simulink model "AME556_Project_Task4_v2"  (R2024b)
settings: Solver=VariableStepAuto  StartTime=0.0  StopTime=5  FixedStep=0.0005  RelTol=1e-3  AbsTol=1e-3
InitFcn:
  | global params;
  | 
  | % Mass and geometry
  | params.m = 0.25;
  | params.l = 0.22;
  | params.mb = 8;
  | params.a = 0.25;
  | params.b = 0.15;
  | params.g = [0; 9.81; 0];
  | 
  | % Moment of inerita
  | Il_zz = params.m * params.l^2 / 12;
  | Ib_xx = params.mb * params.a^2 / 12;
  | Ib_yy = params.mb * params.b^2 / 12;
  | Ib_zz = params.mb * (params.a^2 + params.b^2) / 12;
  | params.Ib = diag([Ib_xx Ib_yy Ib_zz]);
  | 
  | % Spatial contact force parameters
  | Kp_g = 1e5;
  | Kd_g = 1e3;
  | 
  | % Ground contact positions
  | params.P1 = [0.0197; 0.0022; 0];
  | params.P2 = [0.1838; 0.0041; 0];
  | 
  | % State variables
  | q0 = [0.1; 0.45; 0; -pi/3; pi/2; -pi/6; pi/2]; % Initial states (before landing)
  | params.p_d = [0; 0.5; 0]; % Desired positions (after standing): [x_d; y_d; z_d];
  | params.theta_d = 0; % Desired angle
values from neighbouring files (symbols this model uses):
  dt = 0.04    [AME556_Project_Task4_Setup.m]
  l = 2    [AME556_Project_Task4_Setup.m]
  N = 10    [AME556_Project_Task4_Setup.m]
undefined symbols (not defined in the file or in its folder): P1_world0, P2_world0, X, Y, Z
libraries: sm_lib x37, nesl_utility x23
(part 2 of 2)

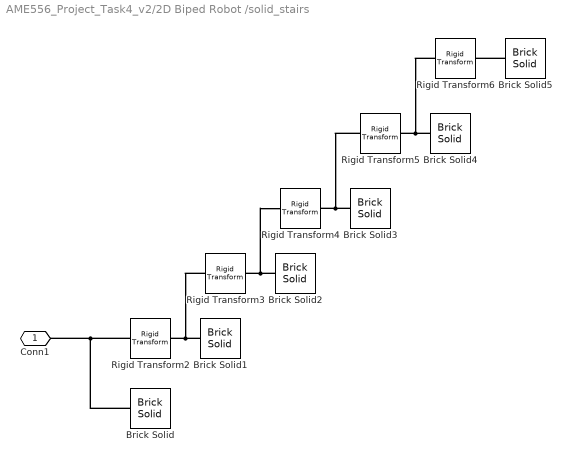
== system AME556_Project_Task4_v2/2D Biped Robot /solid_stairs ==
  Brick Solid : sm_lib/Body Elements/Brick Solid  BrickDimensions=[x_grid(end) y_grid(end) 0.1 ]  BrickDimensionsUnits=m  ExportEntireGeometry=off  InertiaType=CalculateFromGeometry  BasedOnType=Density  Density=1000  DensityUnits=kg/m^3  Mass=1  MassUnits=kg  CenterOfMass=[0 0 0]  CenterOfMassUnits=m  MomentsOfInertia=[1 1 1]  MomentsOfInertiaUnits=kg*m^2  ProductsOfInertia=[0 0 0]  ProductsOfInertiaUnits=kg*m^2  GraphicType=FromGeometry  MarkerShape=Sphere  MarkerSize=10  GraphicVisPropType=SimpleVisualProperties  GraphicDiffuseColor=stairsColor  GraphicOpacity=1  GraphicSpecularColor=[0.5 0.5 0.5 1.0]  GraphicAmbientColor=[0.15 0.15 0.15 1.0]  GraphicEmissiveColor=[0.0 0.0 0.0 1.0]  GraphicShininess=75  DoExposeReferenceFrame=on  SerializedFrames=<Frames><Frame><Id>Frame1</Id><Value><Name>F1</Name><Origin><Source>GeometricFeature</Source><FeatureName>-x -y +z point</FeatureName></Origin><PrimaryAxis><DefinedDirection>+Z</DefinedDirection><Source>ReferenceFrame</Source><SourceDirection>+Z</SourceDirection><FeatureName></FeatureName></PrimaryAxis><SecondaryAxis><DefinedDirection>+X</DefinedDirection><Source>ReferenceFrame</Source><SourceDirection>+X</SourceDirection><FeatureName></FeatureName></SecondaryAxis></Value></Frame></Frames>
  Brick Solid1 : sm_lib/Body Elements/Brick Solid  BrickDimensions=[x_grid(end) 0.8+l 0.1 ]  BrickDimensionsUnits=m  ExportEntireGeometry=off  InertiaType=CalculateFromGeometry  BasedOnType=Density  Density=1000  DensityUnits=kg/m^3  Mass=1  MassUnits=kg  CenterOfMass=[0 0 0]  CenterOfMassUnits=m  MomentsOfInertia=[1 1 1]  MomentsOfInertiaUnits=kg*m^2  ProductsOfInertia=[0 0 0]  ProductsOfInertiaUnits=kg*m^2  GraphicType=FromGeometry  MarkerShape=Sphere  MarkerSize=10  GraphicVisPropType=SimpleVisualProperties  GraphicDiffuseColor=stairsColor  GraphicOpacity=1  GraphicSpecularColor=[0.5 0.5 0.5 1.0]  GraphicAmbientColor=[0.15 0.15 0.15 1.0]  GraphicEmissiveColor=[0.0 0.0 0.0 1.0]  GraphicShininess=75  DoExposeReferenceFrame=on  SerializedFrames=<Frames><Frame><Id>Frame1</Id><Value><Name>F1</Name><Origin><Source>GeometricFeature</Source><FeatureName>-x -y -z point</FeatureName></Origin><PrimaryAxis><DefinedDirection>+Z</DefinedDirection><Source>ReferenceFrame</Source><SourceDirection>+Z</SourceDirection><FeatureName></FeatureName></PrimaryAxis><SecondaryAxis><DefinedDirection>+X</DefinedDirection><Source>ReferenceFrame</Source><SourceDirection>+X</SourceDirection><FeatureName></FeatureName></SecondaryAxis></Value></Frame></Frames>
  Brick Solid2 : sm_lib/Body Elements/Brick Solid  BrickDimensions=[x_grid(end) 0.6+l 0.1 ]  BrickDimensionsUnits=m  ExportEntireGeometry=off  InertiaType=CalculateFromGeometry  BasedOnType=Density  Density=1000  DensityUnits=kg/m^3  Mass=1  MassUnits=kg  CenterOfMass=[0 0 0]  CenterOfMassUnits=m  MomentsOfInertia=[1 1 1]  MomentsOfInertiaUnits=kg*m^2  ProductsOfInertia=[0 0 0]  ProductsOfInertiaUnits=kg*m^2  GraphicType=FromGeometry  MarkerShape=Sphere  MarkerSize=10  GraphicVisPropType=SimpleVisualProperties  GraphicDiffuseColor=stairsColor  GraphicOpacity=1  GraphicSpecularColor=[0.5 0.5 0.5 1.0]  GraphicAmbientColor=[0.15 0.15 0.15 1.0]  GraphicEmissiveColor=[0.0 0.0 0.0 1.0]  GraphicShininess=75  DoExposeReferenceFrame=on  SerializedFrames=<Frames><Frame><Id>Frame1</Id><Value><Name>F1</Name><Origin><Source>GeometricFeature</Source><FeatureName>-x -y -z point</FeatureName></Origin><PrimaryAxis><DefinedDirection>+Z</DefinedDirection><Source>ReferenceFrame</Source><SourceDirection>+Z</SourceDirection><FeatureName></FeatureName></PrimaryAxis><SecondaryAxis><DefinedDirection>+X</DefinedDirection><Source>ReferenceFrame</Source><SourceDirection>+X</SourceDirection><FeatureName></FeatureName></SecondaryAxis></Value></Frame></Frames>
  Brick Solid3 : sm_lib/Body Elements/Brick Solid  BrickDimensions=[x_grid(end) 0.4+l 0.1 ]  BrickDimensionsUnits=m  ExportEntireGeometry=off  InertiaType=CalculateFromGeometry  BasedOnType=Density  Density=1000  DensityUnits=kg/m^3  Mass=1  MassUnits=kg  CenterOfMass=[0 0 0]  CenterOfMassUnits=m  MomentsOfInertia=[1 1 1]  MomentsOfInertiaUnits=kg*m^2  ProductsOfInertia=[0 0 0]  ProductsOfInertiaUnits=kg*m^2  GraphicType=FromGeometry  MarkerShape=Sphere  MarkerSize=10  GraphicVisPropType=SimpleVisualProperties  GraphicDiffuseColor=stairsColor  GraphicOpacity=1  GraphicSpecularColor=[0.5 0.5 0.5 1.0]  GraphicAmbientColor=[0.15 0.15 0.15 1.0]  GraphicEmissiveColor=[0.0 0.0 0.0 1.0]  GraphicShininess=75  DoExposeReferenceFrame=on  SerializedFrames=<Frames><Frame><Id>Frame1</Id><Value><Name>F1</Name><Origin><Source>GeometricFeature</Source><FeatureName>-x -y -z point</FeatureName></Origin><PrimaryAxis><DefinedDirection>+Z</DefinedDirection><Source>ReferenceFrame</Source><SourceDirection>+Z</SourceDirection><FeatureName></FeatureName></PrimaryAxis><SecondaryAxis><DefinedDirection>+X</DefinedDirection><Source>ReferenceFrame</Source><SourceDirection>+X</SourceDirection><FeatureName></FeatureName></SecondaryAxis></Value></Frame></Frames>
  Brick Solid4 : sm_lib/Body Elements/Brick Solid  BrickDimensions=[x_grid(end) 0.2+l 0.1 ]  BrickDimensionsUnits=m  ExportEntireGeometry=off  InertiaType=CalculateFromGeometry  BasedOnType=Density  Density=1000  DensityUnits=kg/m^3  Mass=1  MassUnits=kg  CenterOfMass=[0 0 0]  CenterOfMassUnits=m  MomentsOfInertia=[1 1 1]  MomentsOfInertiaUnits=kg*m^2  ProductsOfInertia=[0 0 0]  ProductsOfInertiaUnits=kg*m^2  GraphicType=FromGeometry  MarkerShape=Sphere  MarkerSize=10  GraphicVisPropType=SimpleVisualProperties  GraphicDiffuseColor=stairsColor  GraphicOpacity=1  GraphicSpecularColor=[0.5 0.5 0.5 1.0]  GraphicAmbientColor=[0.15 0.15 0.15 1.0]  GraphicEmissiveColor=[0.0 0.0 0.0 1.0]  GraphicShininess=75  DoExposeReferenceFrame=on  SerializedFrames=<Frames><Frame><Id>Frame1</Id><Value><Name>F1</Name><Origin><Source>GeometricFeature</Source><FeatureName>-x -y -z point</FeatureName></Origin><PrimaryAxis><DefinedDirection>+Z</DefinedDirection><Source>ReferenceFrame</Source><SourceDirection>+Z</SourceDirection><FeatureName></FeatureName></PrimaryAxis><SecondaryAxis><DefinedDirection>+X</DefinedDirection><Source>ReferenceFrame</Source><SourceDirection>+X</SourceDirection><FeatureName></FeatureName></SecondaryAxis></Value></Frame></Frames>
  Brick Solid5 : sm_lib/Body Elements/Brick Solid  BrickDimensions=[x_grid(end) l 0.1 ]  BrickDimensionsUnits=m  ExportEntireGeometry=off  InertiaType=CalculateFromGeometry  BasedOnType=Density  Density=1000  DensityUnits=kg/m^3  Mass=1  MassUnits=kg  CenterOfMass=[0 0 0]  CenterOfMassUnits=m  MomentsOfInertia=[1 1 1]  MomentsOfInertiaUnits=kg*m^2  ProductsOfInertia=[0 0 0]  ProductsOfInertiaUnits=kg*m^2  GraphicType=FromGeometry  MarkerShape=Sphere  MarkerSize=10  GraphicVisPropType=SimpleVisualProperties  GraphicDiffuseColor=stairsColor  GraphicOpacity=1  GraphicSpecularColor=[0.5 0.5 0.5 1.0]  GraphicAmbientColor=[0.15 0.15 0.15 1.0]  GraphicEmissiveColor=[0.0 0.0 0.0 1.0]  GraphicShininess=75  DoExposeReferenceFrame=on  SerializedFrames=<Frames><Frame><Id>Frame1</Id><Value><Name>F1</Name><Origin><Source>GeometricFeature</Source><FeatureName>-x -y -z point</FeatureName></Origin><PrimaryAxis><DefinedDirection>+Z</DefinedDirection><Source>ReferenceFrame</Source><SourceDirection>+Z</SourceDirection><FeatureName></FeatureName></PrimaryAxis><SecondaryAxis><DefinedDirection>+X</DefinedDirection><Source>ReferenceFrame</Source><SourceDirection>+X</SourceDirection><FeatureName></FeatureName></SecondaryAxis></Value></Frame></Frames>
  Rigid Transform2 : sm_lib/Frames and Transforms/Rigid Transform  RotationMethod=None  FollAlignAxisA=+X  BaseAlignAxisA=+Z  FollAlignAxisB=+Y  BaseAlignAxisB=+X  RotationStandardAxis=+Z  RotationAngle=0  RotationAngleUnits=deg  RotationArbitraryAxis=[0 0 1]  RotationSequenceAxes=FollowerAxes  RotationSequence=XYX  RotationSequenceAngles=[0 0 0]  RotationSequenceAnglesUnits=deg  RotationMatrix=[1 0 0;0 1 0;0 0 1]  Quaternion=[1 0 0 0]  TranslationMethod=StandardAxis  TranslationCartesianOffset=[0 0 0]  TranslationCartesianOffsetUnits=m  TranslationStandardAxis=+Y  TranslationStandardOffset=l  TranslationStandardOffsetUnits=m  TranslationROffset=0  TranslationROffsetUnits=m  TranslationThetaOffset=0  TranslationThetaOffsetUnits=deg  TranslationZOffset=0  TranslationZOffsetUnits=m
  Rigid Transform{3..6} (4 alike) : sm_lib/Frames and Transforms/Rigid Transform  RotationMethod=None  FollAlignAxisA=+X  BaseAlignAxisA=+Z  FollAlignAxisB=+Y  BaseAlignAxisB=+X  RotationStandardAxis=+Z  RotationAngle=0  RotationAngleUnits=deg  RotationArbitraryAxis=[0 0 1]  RotationSequenceAxes=FollowerAxes  RotationSequence=XYX  RotationSequenceAngles=[0 0 0]  RotationSequenceAnglesUnits=deg  RotationMatrix=[1 0 0;0 1 0;0 0 1]  Quaternion=[1 0 0 0]  TranslationMethod=Cartesian  TranslationCartesianOffset=[0 0.2 0.1]  TranslationCartesianOffsetUnits=m  TranslationStandardAxis=+Y  TranslationStandardOffset=l  TranslationStandardOffsetUnits=m  TranslationROffset=0  TranslationROffsetUnits=m  TranslationThetaOffset=0  TranslationThetaOffsetUnits=deg  TranslationZOffset=0  TranslationZOffsetUnits=m
  Conn1 : PMIOPort  Side=Left
  connections:
  Brick Solid3/LConn1 -- Rigid Transform5/LConn1 -- Rigid Transform4/RConn1
  Brick Solid2/LConn1 -- Rigid Transform4/LConn1 -- Rigid Transform3/RConn1
  Brick Solid4/LConn1 -- Rigid Transform6/LConn1 -- Rigid Transform5/RConn1
  Brick Solid/LConn1 -- Conn1/RConn1 -- Rigid Transform2/LConn1
  Brick Solid1/LConn1 -- Rigid Transform3/LConn1 -- Rigid Transform2/RConn1
  Brick Solid5/LConn1 -- Rigid Transform6/RConn1

== matlab function AME556_Project_Task4_v2/MATLAB Function ==
  data: tau_unsaturated input; tau_saturated output; saturateSwitch input
function tau_saturated = tau_saturation(tau_unsaturated, saturateSwitch)
    if saturateSwitch == 1
        tau_limits = [30, 60, 30, 60];
    
        tau_saturated = tau_unsaturated;
    
        for i = 1:length(tau_unsaturated)
            if tau_unsaturated(i) > tau_limits(i)
                tau_saturated(i) = tau_limits(i);
                warning('Tau %d (%.2f) is saturated to %d', i, tau_unsaturated(i), tau_limits(i));
            elseif tau_unsaturated(i) < -tau_limits(i)
                tau_saturated(i) = -tau_limits(i);
                warning('Tau %d (%.2f) is saturated to -%d', i, tau_unsaturated(i), tau_limits(i));
            end
        end
    else
        tau_saturated = tau_unsaturated;
    end
end

== matlab function AME556_Project_Task4_v2/Controller/Condensed MPC Controller ==
  data: p input; theta input; dp input; dtheta input; qs input; tau output; P1 input; P2 input; dP1 input; dP2 input; N input; dt input; t input
%% Function: Low Level Control

function tau = lowLevelControl(p, theta, dp, dtheta, qs, P1, P2, dP1, dP2, N, dt, t)

con = gaitSchedule(N, dt, t);
F = condensed_mpc_controller(p, theta, dp, dtheta, P1, P2, N, dt, t, con);
J = jacobianFcn(theta, qs);

tau = zeros(4, 1);
if con(1, 1) && con(2, 1)
    tau = -J' * F;
elseif con(1, 1) && ~con(2, 1)
    F_swing = swingLegControl(p, dp, P2, dP2, N, dt, t);
    F_new = [F(1: 2); -F_swing];
    tau = -J' * F_new;
elseif con(2, 1) && ~con(1, 1)
    F_swing = swingLegControl(p, dp, P1, dP1, N, dt, t);
    F_new = [-F_swing; F(3: 4)];
    tau = -J' * F_new;    
end

end

%% Function: Condensed MPC Controller

function F = condensed_mpc_controller(p, theta, dp, dtheta, P1, P2, N, dt, t, con)

% Parameters
mt = 8;
a = 0.25;
b = 0.15;
g = [0; 9.81; 0];
Ib_zz = mt * (a^2 + b^2) / 12;

numStates = 7;
numCtrls = 4;
Q = diag([200 200 800 30 10 10 0]);
R = 0.0001*eye(numCtrls);

% q = [x; y; z; R1; dx; dy; dz; wbx; wby; wbz];
% X = [x; y; theta; dx; dy; dtheta; g];
X = zeros(numStates, 1);
X(1: 2) = p;
X(3) = theta;
X(4: 5) = dp;
X(6) = dtheta;
X(7) = g(2);

% Desired states
X_d = getXd(p);
% X_d = [0.5*t; 0.45; 0; 0.5; 0; 0; g(2)];

% Reference Trajectory
X_ref = getReferenceTrajectory(dt, N, p, theta, dp, dtheta, X_d);
y = reshape(X_ref, [numStates*N 1]);

r1 = P1 - p;
r2 = P2 - p;

% Linearized system (A, B)
A = [zeros(3)   eye(3)    zeros(3,1);
     zeros(3, numStates-1) [0; -1; 0];
     zeros(1, numStates)];

B = [zeros(3, numCtrls);
     eye(2)/mt eye(2)/mt;
     -r1(2)/Ib_zz r1(1)/Ib_zz -r2(2)/Ib_zz r2(1)/Ib_zz;
     zeros(1, numCtrls)];

% Discrete-time system matrices (Ak, Bk)
Ak = A * dt + eye(size(A, 1));
Bk = B * dt;

% Aqp
Aqp = [];
for i = 1: N
    Aqp = [Aqp; mpower(Ak, i)];
end

% bqp
Bqp = repmat(zeros(size(Bk)), N, N);
for i = 0: N-1
    element = mpower(Ak, i) * Bk;
    Bqp = Bqp + kron(diag(ones(1, N - i), -i), element);
end

% Condensation
L = kron(eye(N), Q);
K = kron(eye(N), R);

% Optimization weights (H, f)
H = 2*(Bqp'*L*Bqp + K);
f = 2*Bqp'*L*(Aqp*X - y);

% Inequality constraints (A_ineq, b_ineq)
Aineq_mu = kron(eye(2), [1 -0.7; -1 -0.7]);
Aineq_mu_N = kron(eye(N), Aineq_mu);
Aineq_F = kron(eye(2), [0 1; 0 -1]);
Aineq_F_N = kron(eye(N), Aineq_F);
Aineq = [Aineq_mu_N; Aineq_F_N];

bineq_mu = repmat([0; 0; 0; 0], N, 1);
bineq_f = [];
for i = 1: N
    bineq_f = [bineq_f; [250; -10]*con(1, i); [250; -10]*con(2, i)];
end
bineq = [bineq_mu; bineq_f];

% Initial guess
u0 = zeros(length(f), 1);

% Quadratic programming
options = optimoptions('quadprog', 'Algorithm', 'active-set', 'Display', 'off');
u_mpc = quadprog(H, f, Aineq, bineq, [], [], [], [], u0, options);

% Force inputs
F = u_mpc(1: numCtrls);

end

%% Function: Get X_desired
function X_d = getXd(p)
y_d = 0.45;
g = [0; 9.81; 0];
l = 2;

    X_d = [0; y_d; 0; 0; 0; 0; g(2)];

end

%% Function: Get Reference Geometry

function X_ref = getReferenceTrajectory(dt, N, p, theta, dp, dtheta, X_d)

X = [p; theta; dp; dtheta; 9.81];
X_ref = repmat(X, 1, N);

for i = 1: 3
    for k = 2: N
        if X_d(i + 3) ~= 0
            X_ref(i, k) = X(i) + X_d(i+3)*((k-1)*dt);
        else
            X_ref(i, k) = X_d(i);
        end
    end
end

end

%% Function: Swing Leg Control

function F_swing = swingLegControl(p, dp, P, dP, N, dt, t)

% Leg swing height
swingHeight = 0.15;

Kp = diag([200 300]);
Kd = eye(2)*5;
Kv = 0.08;

X_d = getXd(p);

ts = rem(t, N*dt/2);

% Desired leg positions
Px_d = p(1) + (1/2)*(N/2*dt)*dp(1) - Kv * (X_d(4) - dp(1)); % N/2*dt: swinging time
Py_d = swingHeight * sin(pi*ts/(N*dt/2));

F_swing = Kp*([Px_d; Py_d] - P) + Kd*(0 - dP);

end

%% Function: Jacobian Function
% Convert contact forces to joint torques

function J = jacobianFcn(theta, qs)

l = 0.22;

q1 = qs(1); q2 = qs(2); q3 = qs(3); q4 = qs(4);

J = [l*cos(q1 + q2 + theta) + l*cos(q1 + theta), l*cos(q1 + q2 + theta),                                          0,                      0;
     l*sin(q1 + q2 + theta) + l*sin(q1 + theta), l*sin(q1 + q2 + theta),                                          0,                      0;
                                              0,                      0, l*cos(q3 + q4 + theta) + l*cos(q3 + theta), l*cos(q3 + q4 + theta);
                                              0,                      0, l*sin(q3 + q4 + theta) + l*sin(q3 + theta), l*sin(q3 + q4 + theta)];

end

%% Function: Gait Schedule
% Generate gait schedule based on walking phase

function sigma = gaitSchedule(N, dt, t)

phase = floor(t/dt);
k = rem(phase, N);

sigma_l0 = [ones(1, N/2) zeros(1, N/2)];
sigma_r0 = [zeros(1, N/2) ones(1, N/2)];

if k ~= 0
    sigma_l = [sigma_l0(k+1: N) sigma_l0(1: k)];
    sigma_r = [sigma_r0(k+1: N) sigma_r0(1: k)];
else
    sigma_l = sigma_l0;
    sigma_r = sigma_r0;
end

sigma = [sigma_l; sigma_r];

end
